simulink model "controlmodel"  (R2016a)
settings: Solver=ode45  StartTime=0.0  StopTime=12.0  RelTol=1e-3
values from neighbouring files (symbols this model uses):
  gainBFL = 1    [LoadModel_dampedTM.m]
  gainBFP = 1    [LoadModel_dampedTM.m]
  gainBFR = 1    [LoadModel_dampedTM.m]
  gainBFT = 1    [LoadModel_dampedTM.m]
  gainBFV = 1    [LoadModel_dampedTM.m]
  gainBFY = 1    [LoadModel_dampedTM.m]
  gainGASBF = 1    [LoadModel_dampedTM.m]
  gainGASF0 = 1    [LoadModel_dampedTM.m]
  gainGASF1 = 1    [LoadModel_dampedTM.m]
  gainGASF2 = 1    [LoadModel_dampedTM.m]
  gainGASF3 = 1    [LoadModel_dampedTM.m]
  gainIML = 1    [LoadModel_dampedTM.m]
  gainIMP = 1    [LoadModel_dampedTM.m]
  gainIMR = 1    [LoadModel_dampedTM.m]
  gainIMT = 1    [LoadModel_dampedTM.m]
  gainIMV = 1    [LoadModel_dampedTM.m]
  gainIMY = 1    [LoadModel_dampedTM.m]
  gainIPL = 1    [LoadModel_dampedTM.m]
  gainIPT = 1    [LoadModel_dampedTM.m]
  gainIPY = 1    [LoadModel_dampedTM.m]
  gainLOCK_IML = 1    [LoadModel_dampedTM.m]
  gainLOCK_IMP = 1    [LoadModel_dampedTM.m]
  gainLOCK_IMY = 1    [LoadModel_dampedTM.m]
  gainMNL = 1    [LoadModel_dampedTM.m]
  gainMNLOCK_L = 1    [LoadModel_dampedTM.m]
  gainMNLOCK_P = 1    [LoadModel_dampedTM.m]
  gainMNLOCK_Y = 1    [LoadModel_dampedTM.m]
  gainMNP = 1    [LoadModel_dampedTM.m]
  gainMNR = 1    [LoadModel_dampedTM.m]
  gainMNT = 1    [LoadModel_dampedTM.m]
  gainMNV = 1    [LoadModel_dampedTM.m]
  gainMNY = 1    [LoadModel_dampedTM.m]
  gainOL_MNP = 1    [LoadModel_dampedTM.m]
  gainOL_MNY = 1    [LoadModel_dampedTM.m]
  gainTML = 1    [LoadModel_dampedTM.m]
  gainTML_LOCK = 0    [LoadModel_dampedTM.m]
  gainTMOL_IML = 1    [LoadModel_dampedTM.m]
  gainTMOL_IMP = 1    [LoadModel_dampedTM.m]
  gainTMOL_IMY = 1    [LoadModel_dampedTM.m]
  gainTMOL_MNL = 1    [LoadModel_dampedTM.m]
  gainTMOL_MNP = 1    [LoadModel_dampedTM.m]
  gainTMOL_MNY = 1    [LoadModel_dampedTM.m]
  gainTMP = 1    [LoadModel_dampedTM.m]
  gainTMY = 1    [LoadModel_dampedTM.m]
  Kopt_angle = 0.1    [LoadModel_dampedTM.m]
  Kopt_len = 0.1    [LoadModel_dampedTM.m]
  optic = 'ETMX'    [LoadModel_dampedTM.m]
undefined symbols (not defined in the file or in its folder): cMat_BF, cMat_IM, cMat_MN, cMat_TM, Filt, gain_actBFGAS, gain_actBFL, gain_actBFP, gain_actBFR, gain_actBFT, gain_actBFV, gain_actBFY, gain_actF0GAS, gain_actF1GAS, gain_actF2GAS, gain_actF3GAS, gain_actIML, gain_actIMP, gain_actIMR, gain_actIMT, gain_actIMV, gain_actIMY, gain_actIPL, gain_actIPT, gain_actIPY, gain_actMNL, gain_actMNP, gain_actMNR, gain_actMNT, gain_actMNV, gain_actMNY, gain_actTML, gain_actTMP, gain_actTMY, SW, sys1
libraries: cstblocks x49, LiveParts x49
(part 1 of 3)
settings Model: Creator=kokioktm  LastModifiedBy=controls
settings DataIOCC: LimitDataPoints=on  SaveFormat=Array
settings DebuggingCC: SolverPrmCheckMsg=warning
settings HardwareCC: ProdBitPerPointer=32  ProdLargestAtomicFloat=None  ProdIntDivRoundTo=Undefined  ProdEndianess=Unspecified  ProdWordSize=32  ProdHWDeviceType=32-bit Generic
settings ModelReferenceCC: PropagateSignalLabelsOutOfModel=off
settings ConfigComp: CovSFcnEnable=off

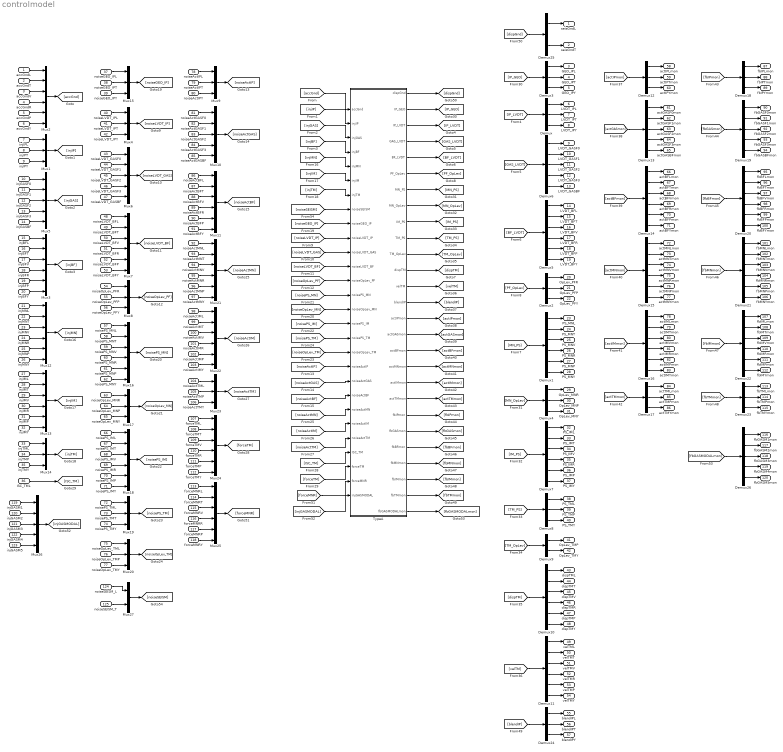
== system controlmodel ==
  accGndL : Inport
  accGndT : Inport  Port=2
  accGndV : Inport  Port=3
  accGndR : Inport  Port=4
  accGndP : Inport  Port=5
  accGndY : Inport  Port=6
  injIPL : Inport  Port=7
  injIPT : Inport  Port=8
  injIPY : Inport  Port=9
  injGASF0 : Inport  Port=10
  injGASF1 : Inport  Port=11
  injGASF2 : Inport  Port=12
  injGASF3 : Inport  Port=13
  injGASBF : Inport  Port=14
  injBFL : Inport  Port=15
  injBFT : Inport  Port=16
  injBFV : Inport  Port=17
  injBFR : Inport  Port=18
  injBFP : Inport  Port=19
  injBFY : Inport  Port=20
  injMNL : Inport  Port=21
  injMNT : Inport  Port=22
  injMNV : Inport  Port=23
  injMNR : Inport  Port=24
  injMNP : Inport  Port=25
  injMNY : Inport  Port=26
  injIML : Inport  Port=27
  injIMT : Inport  Port=28
  injIMV : Inport  Port=29
  injIMR : Inport  Port=30
  injIMP : Inport  Port=31
  injIMY : Inport  Port=32
  injTML : Inport  Port=33
  injTMP : Inport  Port=34
  injTMY : Inport  Port=35
  ISC_TML : Inport  Port=36
  noiseGEO_IPL : Inport  Port=37
  noiseGEO_IPT : Inport  Port=38
  noiseGEO_IPY : Inport  Port=39
  noiseLVDT_IPL : Inport  Port=40
  noiseLVDT_IPT : Inport  Port=41
  noiseLVDT_IPY : Inport  Port=42
  noiseLVDT_GASF0 : Inport  Port=43
  noiseLVDT_GASF1 : Inport  Port=44
  noiseLVDT_GASF2 : Inport  Port=45
  noiseLVDT_GASF3 : Inport  Port=46
  noiseLVDT_GASBF : Inport  Port=47
  noiseLVDT_BFL : Inport  Port=48
  noiseLVDT_BFT : Inport  Port=49
  noiseLVDT_BFV : Inport  Port=50
  noiseLVDT_BFR : Inport  Port=51
  noiseLVDT_BFP : Inport  Port=52
  noiseLVDT_BFY : Inport  Port=53
  noiseOpLev_PFR : Inport  Port=54
  noiseOpLev_PFP : Inport  Port=55
  noiseOpLev_PFY : Inport  Port=56
  noisePS_MNL : Inport  Port=57
  noisePS_MNT : Inport  Port=58
  noisePS_MNV : Inport  Port=59
  noisePS_MNR : Inport  Port=60
  noisePS_MNP : Inport  Port=61
  noisePS_MNY : Inport  Port=62
  noiseOpLev_MNR : Inport  Port=63
  noiseOpLev_MNP : Inport  Port=64
  noiseOpLev_MNY : Inport  Port=65
  noisePS_IML : Inport  Port=66
  noisePS_IMT : Inport  Port=67
  noisePS_IMV : Inport  Port=68
  noisePS_IMR : Inport  Port=69
  noisePS_IMP : Inport  Port=70
  noisePS_IMY : Inport  Port=71
  noisePS_TML : Inport  Port=72
  noisePS_TMT : Inport  Port=73
  noisePS_TMY : Inport  Port=74
  noiseOpLev_TML : Inport  Port=75
  noiseOpLev_TMP : Inport  Port=76
  noiseOpLev_TMY : Inport  Port=77
  noiseActIPL : Inport  Port=78
  noiseActIPT : Inport  Port=79
  noiseActIPY : Inport  Port=80
  noiseActGASF0 : Inport  Port=81
  noiseActGASF1 : Inport  Port=82
  noiseActGASF2 : Inport  Port=83
  noiseActGASF3 : Inport  Port=84
  noiseActGASBF : Inport  Port=85
  noiseActBFL : Inport  Port=86
  noiseActBFT : Inport  Port=87
  noiseActBFV : Inport  Port=88
  noiseActBFR : Inport  Port=89
  noiseActBFP : Inport  Port=90
  noiseActBFY : Inport  Port=91
  noiseActMNL : Inport  Port=92
  noiseActMNT : Inport  Port=93
  noiseActMNV : Inport  Port=94
  noiseActMNR : Inport  Port=95
  noiseActMNP : Inport  Port=96
  noiseActMNY : Inport  Port=97
  noiseActIML : Inport  Port=98
  noiseActIMT : Inport  Port=99
  noiseActIMV : Inport  Port=100
  noiseActIMR : Inport  Port=101
  noiseActIMP : Inport  Port=102
  noiseActIMY : Inport  Port=103
  noiseActTML : Inport  Port=104
  noiseActTMP : Inport  Port=105
  noiseActTMY : Inport  Port=106
  forceTML : Inport  Port=107
  forceTMT : Inport  Port=108
  forceTMV : Inport  Port=109
  forceTMR : Inport  Port=110
  forceTMP : Inport  Port=111
  forceTMY : Inport  Port=112
  forceMNRL : Inport  Port=113
  forceMNRT : Inport  Port=114
  forceMNRV : Inport  Port=115
  forceMNRR : Inport  Port=116
  forceMNRP : Inport  Port=117
  forceMNRY : Inport  Port=118
  injGASM1 : Inport  Port=119
  injGASM2 : Inport  Port=120
  injGASM3 : Inport  Port=121
  injGASM4 : Inport  Port=122
  injGASM5 : Inport  Port=123
  noiseSEISM_L : Inport  Port=124
  noiseSEISM_T : Inport  Port=125
  Demux{,2..4,8,12,17..18,23..24} (10 alike) : Demux  Outputs=3
  Demux{1,5,7,10..11,14..16,20..22} (11 alike) : Demux  Outputs=6
  Demux{6,13,19,26} (4 alike) : Demux  Outputs=5
  Demux25 : Demux  Outputs=2
  Demux9 : Demux  Outputs=2
  Mux{1,4,8..9,14..15,17,19..20,23} (10 alike) : Mux  Inputs=3
  Mux{5..6,10,26} (4 alike) : Mux  Inputs=5
  Mux{2..3,7,11..13,16,18,21..22,24..25} (12 alike) : Mux  Inputs=6
  Mux27 : Mux  Inputs=2
  TypeA : Subsystem
  seisGndL : Outport
  seisGndT : Outport  Port=2
  GEO_IPL : Outport  Port=3
  GEO_IPT : Outport  Port=4
  GEO_IPY : Outport  Port=5
  LVDT_IPL : Outport  Port=6
  LVDT_IPT : Outport  Port=7
  LVDT_IPY : Outport  Port=8
  LVDT_GASF0 : Outport  Port=9
  LVDT_GASF1 : Outport  Port=10
  LVDT_GASF2 : Outport  Port=11
  LVDT_GASF3 : Outport  Port=12
  LVDT_GASBF : Outport  Port=13
  LVDT_BFL : Outport  Port=14
  LVDT_BFT : Outport  Port=15
  LVDT_BFV : Outport  Port=16
  LVDT_BFR : Outport  Port=17
  LVDT_BFP : Outport  Port=18
  LVDT_BFY : Outport  Port=19
  OpLev_PFR : Outport  Port=20
  OpLev_PFP : Outport  Port=21
  OpLev_PFY : Outport  Port=22
  PS_MNL : Outport  Port=23
  PS_MNT : Outport  Port=24
  PS_MNV : Outport  Port=25
  PS_MNR : Outport  Port=26
  PS_MNP : Outport  Port=27
  PS_MNY : Outport  Port=28
  OpLev_MNR : Outport  Port=29
  OpLev_MNP : Outport  Port=30
  OpLev_MNY : Outport  Port=31
  PS_IML : Outport  Port=32
  PS_IMT : Outport  Port=33
  PS_IMV : Outport  Port=34
  PS_IMR : Outport  Port=35
  PS_IMP : Outport  Port=36
  PS_IMY : Outport  Port=37
  PS_TML : Outport  Port=38
  PS_TMP : Outport  Port=39
  PS_TMY : Outport  Port=40
  OpLev_TMP : Outport  Port=41
  OpLev_TMY : Outport  Port=42
  dispTML : Outport  Port=43
  dispTMT : Outport  Port=44
  dispTMV : Outport  Port=45
  dispTMR : Outport  Port=46
  dispTMP : Outport  Port=47
  dispTMY : Outport  Port=48
  velTML : Outport  Port=49
  velTMT : Outport  Port=50
  velTMV : Outport  Port=51
  velTMR : Outport  Port=52
  velTMP : Outport  Port=53
  velTMY : Outport  Port=54
  blendIPL : Outport  Port=55
  blendIPT : Outport  Port=56
  blendIPY : Outport  Port=57
  actIPLmon : Outport  Port=58
  actIPTmon : Outport  Port=59
  actIPYmon : Outport  Port=60
  actGASF0mon : Outport  Port=61
  actGASF1mon : Outport  Port=62
  actGASF2mon : Outport  Port=63
  actGASF3mon : Outport  Port=64
  actGASBFmon : Outport  Port=65
  actBFLmon : Outport  Port=66
  actBFTmon : Outport  Port=67
  actBFVmon : Outport  Port=68
  actBFRmon : Outport  Port=69
  actBFPmon : Outport  Port=70
  actBFYmon : Outport  Port=71
  actMNLmon : Outport  Port=72
  actMNTmon : Outport  Port=73
  actMNVmon : Outport  Port=74
  actMNRmon : Outport  Port=75
  actMNPmon : Outport  Port=76
  actMNYmon : Outport  Port=77
  actIMLmon : Outport  Port=78
  actIMTmon : Outport  Port=79
  actIMVmon : Outport  Port=80
  actIMRmon : Outport  Port=81
  actIMPmon : Outport  Port=82
  actIMYmon : Outport  Port=83
  actTMLmon : Outport  Port=84
  actTMPmon : Outport  Port=85
  actTMYmon : Outport  Port=86
  fbIPLmon : Outport  Port=87
  fbIPTmon : Outport  Port=88
  fbIPYmon : Outport  Port=89
  fbGASF0mon : Outport  Port=90
  fbGASF1mon : Outport  Port=91
  fbGASF2mon : Outport  Port=92
  fbGASF3mon : Outport  Port=93
  fbGASBFmon : Outport  Port=94
  fbBFLmon : Outport  Port=95
  fbBFTmon : Outport  Port=96
  fbBFVmon : Outport  Port=97
  fbBFRmon : Outport  Port=98
  fbBFPmon : Outport  Port=99
  fbBFYmon : Outport  Port=100
  fbMNLmon : Outport  Port=101
  fbMNTmon : Outport  Port=102
  fbMNVmon : Outport  Port=103
  fbMNRmon : Outport  Port=104
  fbMNPmon : Outport  Port=105
  fbMNYmon : Outport  Port=106
  fbIMLmon : Outport  Port=107
  fbIMTmon : Outport  Port=108
  fbIMVmon : Outport  Port=109
  fbIMRmon : Outport  Port=110
  fbIMPmon : Outport  Port=111
  fbIMYmon : Outport  Port=112
  fbTMLmon : Outport  Port=113
  fbTMPmon : Outport  Port=114
  fbTMYmon : Outport  Port=115
  fbGASM1mon : Outport  Port=116
  fbGASM2mon : Outport  Port=117
  fbGASM3mon : Outport  Port=118
  fbGASM4mon : Outport  Port=119
  fbGASM5mon : Outport  Port=120
  wires:
  [accGnd] -> TypeA/1(accGnd)
  accGndT/1 -> Mux2/2
  accGndL/1 -> Mux2/1
  accGndV/1 -> Mux2/3
  accGndR/1 -> Mux2/4
  accGndP/1 -> Mux2/5
  accGndY/1 -> Mux2/6
  Mux2/1 -> [accGnd]
  injIPL/1 -> Mux1/1
  injIPT/1 -> Mux1/2
  injIPY/1 -> Mux1/3
  Mux1/1 -> [injIP]
  [injIP] -> TypeA/2(injIP)
  injGASF0/1 -> Mux5/1
  injGASF1/1 -> Mux5/2
  injGASF2/1 -> Mux5/3
  injGASF3/1 -> Mux5/4
  injGASBF/1 -> Mux5/5
  Mux5/1 -> [injGAS]
  [injGAS] -> TypeA/3(injGAS)
  injBFT/1 -> Mux3/2
  injBFL/1 -> Mux3/1
  injBFV/1 -> Mux3/3
  injBFR/1 -> Mux3/4
  injBFP/1 -> Mux3/5
  injBFY/1 -> Mux3/6
  Mux3/1 -> [injBF]
  [injBF] -> TypeA/4(injBF)
  TypeA/3(IP_LVDT) -> [IP_LVDT]
  TypeA/4(GAS_LVDT) -> [GAS_LVDT]
  TypeA/5(BF_LVDT) -> [BF_LVDT]
  TypeA/12(dispTM) -> [dispTM]
  TypeA/6(PF_OpLev) -> [PF_OpLev]
  [IP_LVDT] -> Demux/1
  Demux/1 -> LVDT_IPL/1
  Demux/2 -> LVDT_IPT/1
  Demux/3 -> LVDT_IPY/1
  [GAS_LVDT] -> Demux6/1
  Demux6/1 -> LVDT_GASF0/1
  Demux6/2 -> LVDT_GASF1/1
  Demux6/3 -> LVDT_GASF2/1
  Demux6/4 -> LVDT_GASF3/1
  Demux6/5 -> LVDT_GASBF/1
  [BF_LVDT] -> Demux5/1
  Demux5/1 -> LVDT_BFL/1
  Demux5/2 -> LVDT_BFT/1
  Demux5/3 -> LVDT_BFV/1
  Demux5/4 -> LVDT_BFR/1
  Demux5/5 -> LVDT_BFP/1
  Demux5/6 -> LVDT_BFY/1
  Demux1/1 -> PS_MNL/1
  Demux1/2 -> PS_MNT/1
  Demux1/3 -> PS_MNV/1
  Demux1/4 -> PS_MNR/1
  Demux1/5 -> PS_MNP/1
  Demux1/6 -> PS_MNY/1
  [MN_PS] -> Demux1/1
  [PF_OpLev] -> Demux2/1
  Demux2/2 -> OpLev_PFP/1
  Demux2/3 -> OpLev_PFY/1
  noiseLVDT_IPL/1 -> Mux4/1
  noiseLVDT_IPT/1 -> Mux4/2
  noiseLVDT_IPY/1 -> Mux4/3
  Mux4/1 -> [noiseLVDT_IP]
  noiseLVDT_GASF0/1 -> Mux6/1
  noiseLVDT_GASF1/1 -> Mux6/2
  noiseLVDT_GASF2/1 -> Mux6/3
  noiseLVDT_GASF3/1 -> Mux6/4
  noiseLVDT_GASBF/1 -> Mux6/5
  Mux6/1 -> [noiseLVDT_GAS]
  noiseLVDT_BFT/1 -> Mux7/2
  noiseLVDT_BFL/1 -> Mux7/1
  noiseLVDT_BFV/1 -> Mux7/3
  noiseLVDT_BFR/1 -> Mux7/4
  noiseLVDT_BFP/1 -> Mux7/5
  noiseLVDT_BFY/1 -> Mux7/6
  Mux7/1 -> [noiseLVDT_BF]
  noiseOpLev_PFR/1 -> Mux8/1
  noiseOpLev_PFP/1 -> Mux8/2
  Mux8/1 -> [noiseOpLev_PF]
  [noiseLVDT_IP] -> TypeA/10(noiseLVDT_IP)
  [noiseLVDT_GAS] -> TypeA/11(noiseLVDT_GAS)
  [noiseOpLev_PF] -> TypeA/13(noiseOpLev_PF)
  [noiseLVDT_BF] -> TypeA/12(noiseLVDT_BF)
  noiseActIPL/1 -> Mux9/1
  noiseActIPT/1 -> Mux9/2
  noiseActIPY/1 -> Mux9/3
  Mux9/1 -> [noiseActIP]
  noiseActGASF0/1 -> Mux10/1
  noiseActGASF1/1 -> Mux10/2
  noiseActGASF2/1 -> Mux10/3
  noiseActGASF3/1 -> Mux10/4
  noiseActGASBF/1 -> Mux10/5
  Mux10/1 -> [noiseActGAS]
  noiseActBFT/1 -> Mux11/2
  noiseActBFL/1 -> Mux11/1
  noiseActBFV/1 -> Mux11/3
  noiseActBFR/1 -> Mux11/4
  noiseActBFP/1 -> Mux11/5
  noiseActBFY/1 -> Mux11/6
  Mux11/1 -> [noiseActBF]
  [noiseActGAS] -> TypeA/20(noiseActGAS)
  [noiseActBF] -> TypeA/21(noiseActBF)
  [noiseActIP] -> TypeA/19(noiseActIP)
  [injMN] -> TypeA/5(injMN)
  [injTM] -> TypeA/7(injTM)
  [injIM] -> TypeA/6(injIM)
  injMNT/1 -> Mux12/2
  injMNL/1 -> Mux12/1
  injMNV/1 -> Mux12/3
  injMNR/1 -> Mux12/4
  injMNP/1 -> Mux12/5
  injMNY/1 -> Mux12/6
  Mux12/1 -> [injMN]
  injIMT/1 -> Mux13/2
  injIML/1 -> Mux13/1
  injIMV/1 -> Mux13/3
  injIMR/1 -> Mux13/4
  injIMP/1 -> Mux13/5
  injIMY/1 -> Mux13/6
  Mux13/1 -> [injIM]
  injTML/1 -> Mux14/1
  injTMP/1 -> Mux14/2
  injTMY/1 -> Mux14/3
  Mux14/1 -> [injTM]
  noiseGEO_IPL/1 -> Mux15/1
  noiseGEO_IPT/1 -> Mux15/2
  noiseGEO_IPY/1 -> Mux15/3
  Mux15/1 -> [noiseGEO_IP]
  [noiseGEO_IP] -> TypeA/9(noiseGEO_IP)
  noiseOpLev_PFY/1 -> Mux8/3
  noisePS_MNT/1 -> Mux16/2
  noisePS_MNL/1 -> Mux16/1
  noisePS_MNV/1 -> Mux16/3
  noisePS_MNR/1 -> Mux16/4
  noisePS_MNP/1 -> Mux16/5
  noisePS_MNY/1 -> Mux16/6
  Mux16/1 -> [noisePS_MN]
  noiseOpLev_MNR/1 -> Mux17/1
  noiseOpLev_MNP/1 -> Mux17/2
  Mux17/1 -> [noiseOpLev_MN]
  noiseOpLev_MNY/1 -> Mux17/3
  noisePS_IMT/1 -> Mux18/2
  noisePS_IML/1 -> Mux18/1
  noisePS_IMV/1 -> Mux18/3
  noisePS_IMR/1 -> Mux18/4
  noisePS_IMP/1 -> Mux18/5
  noisePS_IMY/1 -> Mux18/6
  Mux18/1 -> [noisePS_IM]
  noisePS_TML/1 -> Mux19/1
  noisePS_TMT/1 -> Mux19/2
  Mux19/1 -> [noisePS_TM]
  noisePS_TMY/1 -> Mux19/3
  noiseOpLev_TMP/1 -> Mux20/2
  noiseOpLev_TMY/1 -> Mux20/3
  Mux20/1 -> [noiseOpLev_TM]
  [noisePS_MN] -> TypeA/14(noisePS_MN)
  [noisePS_IM] -> TypeA/16(noisePS_IM)
  [noiseOpLev_MN] -> TypeA/15(noiseOpLev_MN)
  [noisePS_TM] -> TypeA/17(noisePS_TM)
  [noiseOpLev_TM] -> TypeA/18(noiseOpLev_TM)
  noiseActMNT/1 -> Mux21/2
  noiseActMNL/1 -> Mux21/1
  noiseActMNV/1 -> Mux21/3
  noiseActMNR/1 -> Mux21/4
  noiseActMNP/1 -> Mux21/5
  noiseActMNY/1 -> Mux21/6
  Mux21/1 -> [noiseActMN]
  noiseActIMT/1 -> Mux22/2
  noiseActIML/1 -> Mux22/1
  noiseActIMV/1 -> Mux22/3
  noiseActIMR/1 -> Mux22/4
  noiseActIMP/1 -> Mux22/5
  noiseActIMY/1 -> Mux22/6
  Mux22/1 -> [noiseActIM]
  noiseActTML/1 -> Mux23/1
  noiseActTMP/1 -> Mux23/2
  noiseActTMY/1 -> Mux23/3
  Mux23/1 -> [noiseActTM]
  forceTMT/1 -> Mux24/2
  forceTML/1 -> Mux24/1
  forceTMV/1 -> Mux24/3
  forceTMR/1 -> Mux24/4
  forceTMP/1 -> Mux24/5
  forceTMY/1 -> Mux24/6
  Mux24/1 -> [forceTM]
  ISC_TML/1 -> [ISC_TM]
  [noiseActMN] -> TypeA/22(noiseActMN)
  [noiseActTM] -> TypeA/24(noiseActTM)
  [noiseActIM] -> TypeA/23(noiseActIM)
  [forceTM] -> TypeA/26(forceTM)
  [ISC_TM] -> TypeA/25(ISC_TM)
  [IP_GEO] -> Demux3/1
  Demux3/1 -> GEO_IPL/1
  Demux3/2 -> GEO_IPT/1
  Demux3/3 -> GEO_IPY/1
  TypeA/2(IP_GEO) -> [IP_GEO]
  Demux2/1 -> OpLev_PFR/1
  TypeA/9(IM_PS) -> [IM_PS]
  TypeA/10(TM_PS) -> [TM_PS]
  TypeA/8(MN_OpLev) -> [MN_OpLev]
  TypeA/7(MN_PS) -> [MN_PS]
  TypeA/11(TM_OpLev) -> [TM_OpLev]
  TypeA/22(fbGASmon) -> [fbGASmon]
  TypeA/16(actGASmon) -> [actGASmon]
  TypeA/21(fbIPmon) -> [fbIPmon]
  TypeA/26(fbTMmon) -> [fbTMmon]
  TypeA/24(fbMNmon) -> [fbMNmon]
  TypeA/15(actIPmon) -> [actIPmon]
  TypeA/19(actIMmon) -> [actIMmon]
  TypeA/14(blendIP) -> [blendIP]
  TypeA/13(velTM) -> [velTM]
  TypeA/25(fbIMmon) -> [fbIMmon]
  TypeA/18(actMNmon) -> [actMNmon]
  TypeA/20(actTMmon) -> [actTMmon]
  TypeA/17(actBFmon) -> [actBFmon]
  TypeA/23(fbBFmon) -> [fbBFmon]
  [MN_OpLev] -> Demux4/1
  Demux4/2 -> OpLev_MNP/1
  Demux4/3 -> OpLev_MNY/1
  Demux4/1 -> OpLev_MNR/1
  Demux7/1 -> PS_IML/1
  Demux7/2 -> PS_IMT/1
  Demux7/3 -> PS_IMV/1
  Demux7/4 -> PS_IMR/1
  Demux7/5 -> PS_IMP/1
  Demux7/6 -> PS_IMY/1
  [IM_PS] -> Demux7/1
  Demux8/1 -> PS_TML/1
  [TM_PS] -> Demux8/1
  Demux8/2 -> PS_TMP/1
  Demux8/3 -> PS_TMY/1
  [TM_OpLev] -> Demux9/1
  Demux9/1 -> OpLev_TMP/1
  Demux9/2 -> OpLev_TMY/1
  Demux10/1 -> dispTML/1
  Demux10/2 -> dispTMT/1
  Demux10/3 -> dispTMV/1
  Demux10/4 -> dispTMR/1
  Demux10/5 -> dispTMP/1
  Demux10/6 -> dispTMY/1
  [dispTM] -> Demux10/1
  Demux11/1 -> velTML/1
  Demux11/2 -> velTMT/1
  Demux11/3 -> velTMV/1
  Demux11/4 -> velTMR/1
  Demux11/5 -> velTMP/1
  Demux11/6 -> velTMY/1
  [velTM] -> Demux11/1
  [actIPmon] -> Demux12/1
  Demux12/1 -> actIPLmon/1
  Demux12/2 -> actIPTmon/1
  Demux12/3 -> actIPYmon/1
  [actGASmon] -> Demux13/1
  Demux13/1 -> actGASF0mon/1
  Demux13/2 -> actGASF1mon/1
  Demux13/3 -> actGASF2mon/1
  Demux13/4 -> actGASF3mon/1
  Demux13/5 -> actGASBFmon/1
  [actBFmon] -> Demux14/1
  Demux14/1 -> actBFLmon/1
  Demux14/2 -> actBFTmon/1
  Demux14/3 -> actBFVmon/1
  Demux14/4 -> actBFRmon/1
  Demux14/5 -> actBFPmon/1
  Demux14/6 -> actBFYmon/1
  [actMNmon] -> Demux15/1
  Demux15/1 -> actMNLmon/1
  Demux15/2 -> actMNTmon/1
  Demux15/3 -> actMNVmon/1
  Demux15/4 -> actMNRmon/1
  Demux15/5 -> actMNPmon/1
  Demux15/6 -> actMNYmon/1
  [actIMmon] -> Demux16/1
  Demux16/1 -> actIMLmon/1
  Demux16/2 -> actIMTmon/1
  Demux16/3 -> actIMVmon/1
  Demux16/4 -> actIMRmon/1
  Demux16/5 -> actIMPmon/1
  Demux16/6 -> actIMYmon/1
  [actTMmon] -> Demux17/1
  Demux17/2 -> actTMPmon/1
  Demux17/3 -> actTMYmon/1
  Demux17/1 -> actTMLmon/1
  [fbIPmon] -> Demux18/1
  Demux18/1 -> fbIPLmon/1
  Demux18/2 -> fbIPTmon/1
  Demux18/3 -> fbIPYmon/1
  [fbGASmon] -> Demux19/1
  Demux19/1 -> fbGASF0mon/1
  Demux19/2 -> fbGASF1mon/1
  Demux19/3 -> fbGASF2mon/1
  Demux19/4 -> fbGASF3mon/1
  Demux19/5 -> fbGASBFmon/1
  [fbBFmon] -> Demux20/1
  Demux20/1 -> fbBFLmon/1
  Demux20/2 -> fbBFTmon/1
  Demux20/3 -> fbBFVmon/1
  Demux20/4 -> fbBFRmon/1
  Demux20/5 -> fbBFPmon/1
  Demux20/6 -> fbBFYmon/1
  [fbMNmon] -> Demux21/1
  Demux21/1 -> fbMNLmon/1
  Demux21/2 -> fbMNTmon/1
  Demux21/3 -> fbMNVmon/1
  Demux21/4 -> fbMNRmon/1
  Demux21/5 -> fbMNPmon/1
  Demux21/6 -> fbMNYmon/1
  [fbIMmon] -> Demux22/1
  Demux22/1 -> fbIMLmon/1
  Demux22/2 -> fbIMTmon/1
  Demux22/3 -> fbIMVmon/1
  Demux22/4 -> fbIMRmon/1
  Demux22/5 -> fbIMPmon/1
  Demux22/6 -> fbIMYmon/1
  [fbTMmon] -> Demux23/1
  Demux23/2 -> fbTMPmon/1
  Demux23/3 -> fbTMYmon/1
  Demux23/1 -> fbTMLmon/1
  Demux24/1 -> blendIPL/1
  [blendIP] -> Demux24/1
  Demux24/2 -> blendIPT/1
  Demux24/3 -> blendIPY/1
  [dispGnd] -> Demux25/1
  Demux25/1 -> seisGndL/1
  Demux25/2 -> seisGndT/1
  TypeA/1(dispGnd) -> [dispGnd]
  forceMNRR/1 -> Mux25/4
  forceMNRP/1 -> Mux25/5
  forceMNRL/1 -> Mux25/1
  forceMNRT/1 -> Mux25/2
  Mux25/1 -> [forceMNR]
  forceMNRV/1 -> Mux25/3
  forceMNRY/1 -> Mux25/6
  [forceMNR] -> TypeA/27(forceMNR)
  noiseOpLev_TML/1 -> Mux20/1
  [injGASMODAL] -> TypeA/28(injGASMODAL)
  injGASM1/1 -> Mux26/1
  injGASM2/1 -> Mux26/2
  injGASM3/1 -> Mux26/3
  injGASM4/1 -> Mux26/4
  injGASM5/1 -> Mux26/5
  Mux26/1 -> [injGASMODAL]
  TypeA/27(fbGASMODALmon) -> [fbGASMODALmon]
  [fbGASMODALmon] -> Demux26/1
  Demux26/1 -> fbGASM1mon/1
  Demux26/2 -> fbGASM2mon/1
  Demux26/3 -> fbGASM3mon/1
  Demux26/4 -> fbGASM4mon/1
  Demux26/5 -> fbGASM5mon/1
  [noiseSEISM] -> TypeA/8(noiseSEISM)
  noiseSEISM_T/1 -> Mux27/2
  Mux27/1 -> [noiseSEISM]
  noiseSEISM_L/1 -> Mux27/1

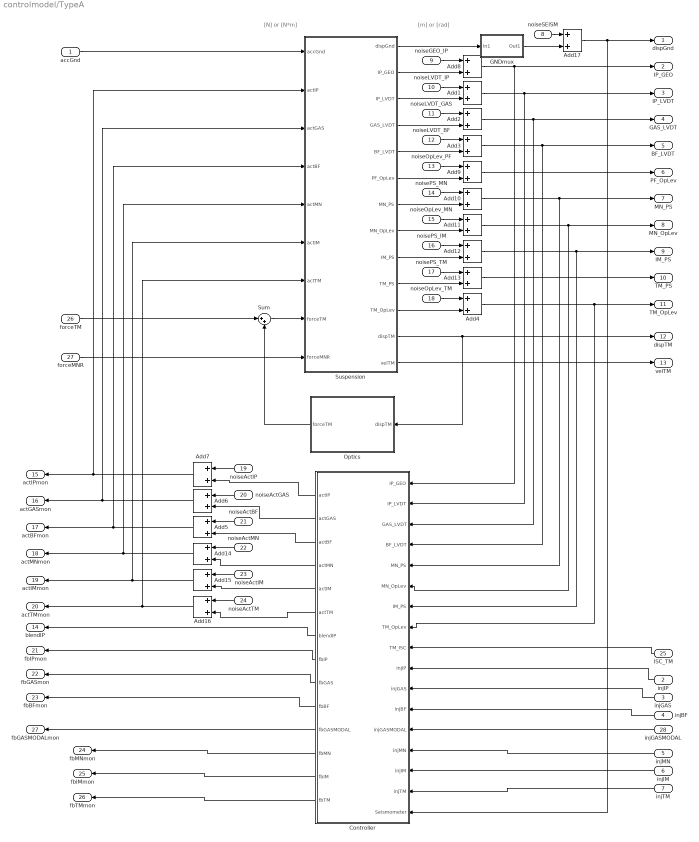
== system controlmodel/TypeA ==
  note: [N] or [N*m]
  note: [m] or [rad]
  accGnd : Inport
  injIP : Inport  Port=2
  injGAS : Inport  Port=3
  injBF : Inport  Port=4
  injMN : Inport  Port=5
  injIM : Inport  Port=6
  injTM : Inport  Port=7
  noiseSEISM : Inport  Port=8
  noiseGEO_IP : Inport  Port=9
  noiseLVDT_IP : Inport  Port=10
  noiseLVDT_GAS : Inport  Port=11
  noiseLVDT_BF : Inport  Port=12
  noiseOpLev_PF : Inport  Port=13
  noisePS_MN : Inport  Port=14
  noiseOpLev_MN : Inport  Port=15
  noisePS_IM : Inport  Port=16
  noisePS_TM : Inport  Port=17
  noiseOpLev_TM : Inport  Port=18
  noiseActIP : Inport  Port=19
  noiseActGAS : Inport  Port=20
  noiseActBF : Inport  Port=21
  noiseActMN : Inport  Port=22
  noiseActIM : Inport  Port=23
  noiseActTM : Inport  Port=24
  ISC_TM : Inport  Port=25
  forceTM : Inport  Port=26
  forceMNR : Inport  Port=27
  injGASMODAL : Inport  Port=28
  Add{1..17} (17 alike) : Sum
  Controller : Subsystem
  GNDmux : Subsystem
  Optics : Subsystem
  Sum : Sum  Inputs=|++
  Suspension : Subsystem
  dispGnd : Outport
  IP_GEO : Outport  Port=2
  IP_LVDT : Outport  Port=3
  GAS_LVDT : Outport  Port=4
  BF_LVDT : Outport  Port=5
  PF_OpLev : Outport  Port=6
  MN_PS : Outport  Port=7
  MN_OpLev : Outport  Port=8
  IM_PS : Outport  Port=9
  TM_PS : Outport  Port=10
  TM_OpLev : Outport  Port=11
  dispTM : Outport  Port=12
  velTM : Outport  Port=13
  blendIP : Outport  Port=14
  actIPmon : Outport  Port=15
  actGASmon : Outport  Port=16
  actBFmon : Outport  Port=17
  actMNmon : Outport  Port=18
  actIMmon : Outport  Port=19
  actTMmon : Outport  Port=20
  fbIPmon : Outport  Port=21
  fbGASmon : Outport  Port=22
  fbBFmon : Outport  Port=23
  fbMNmon : Outport  Port=24
  fbIMmon : Outport  Port=25
  fbTMmon : Outport  Port=26
  fbGASMODALmon : Outport  Port=27
  wires:
  Add1/1 -> IP_LVDT/1, Controller/2(IP_LVDT)
  Add3/1 -> Controller/4(BF_LVDT), BF_LVDT/1
  Add2/1 -> GAS_LVDT/1, Controller/3(GAS_LVDT)
  Add7/1 -> actIPmon/1, Suspension/2(actIP)
  Add5/1 -> actBFmon/1, Suspension/4(actBF)
  Add4/1 -> Controller/8(TM_OpLev), TM_OpLev/1
  accGnd/1 -> Suspension/1(accGnd)
  Add6/1 -> actGASmon/1, Suspension/3(actGAS)
  injGAS/1 -> Controller/11(injGAS)
  injIP/1 -> Controller/10(injIP)
  injBF/1 -> Controller/12(injBF)
  Controller/10(fbBF) -> fbBFmon/1
  Controller/8(fbIP) -> fbIPmon/1
  Controller/9(fbGAS) -> fbGASmon/1
  Suspension/3(IP_LVDT) -> Add1/2
  Suspension/4(GAS_LVDT) -> Add2/2
  Suspension/5(BF_LVDT) -> Add3/2
  Suspension/11(TM_OpLev) -> Add4/2
  noiseLVDT_IP/1 -> Add1/1
  noiseLVDT_GAS/1 -> Add2/1
  noiseLVDT_BF/1 -> Add3/1
  noiseOpLev_TM/1 -> Add4/1
  Controller/3(actBF) -> Add5/2
  Controller/1(actIP) -> Add7/2
  Controller/2(actGAS) -> Add6/2
  noiseActIP/1 -> Add7/1
  noiseActGAS/1 -> Add6/1
  noiseActBF/1 -> Add5/1
  Add8/1 -> Controller/1(IP_GEO), IP_GEO/1
  noiseGEO_IP/1 -> Add8/1
  Suspension/2(IP_GEO) -> Add8/2
  noiseOpLev_PF/1 -> Add9/1
  Suspension/6(PF_OpLev) -> Add9/2
  Add9/1 -> PF_OpLev/1
  noisePS_MN/1 -> Add10/1
  Add10/1 -> Controller/5(MN_PS), MN_PS/1
  noiseOpLev_MN/1 -> Add11/1
  Add11/1 -> Controller/6(MN_OpLev), MN_OpLev/1
  noisePS_IM/1 -> Add12/1
  Add12/1 -> Controller/7(IM_PS), IM_PS/1
  Suspension/8(MN_OpLev) -> Add11/2
  Suspension/7(MN_PS) -> Add10/2
  Suspension/9(IM_PS) -> Add12/2
  noisePS_TM/1 -> Add13/1
  Add13/1 -> TM_PS/1
  Suspension/10(TM_PS) -> Add13/2
  Suspension/13(velTM) -> velTM/1
  injMN/1 -> Controller/14(injMN)
  injTM/1 -> Controller/16(injTM)
  injIM/1 -> Controller/15(injIM)
  ISC_TM/1 -> Controller/9(TM_ISC)
  noiseActMN/1 -> Add14/1
  Add14/1 -> Suspension/5(actMN), actMNmon/1
  Controller/4(actMN) -> Add14/2
  noiseActIM/1 -> Add15/1
  Add15/1 -> Suspension/6(actIM), actIMmon/1
  Controller/5(actIM) -> Add15/2
  noiseActTM/1 -> Add16/1
  Add16/1 -> Suspension/7(actTM), actTMmon/1
  Controller/6(actTM) -> Add16/2
  Controller/7(blendIP) -> blendIP/1
  Controller/14(fbTM) -> fbTMmon/1
  Controller/12(fbMN) -> fbMNmon/1
  Controller/13(fbIM) -> fbIMmon/1
  forceMNR/1 -> Suspension/9(forceMNR)
  injGASMODAL/1 -> Controller/13(injGASMODAL)
  Controller/11(fbGASMODAL) -> fbGASMODALmon/1
  noiseSEISM/1 -> Add17/1
  Add17/1 -> Controller/17(Seismometer), dispGnd/1
  Suspension/12(dispTM) -> Optics/1(dispTM), dispTM/1
  Optics/1(forceTM) -> Sum/2
  forceTM/1 -> Sum/1
  Sum/1 -> Suspension/8(forceTM)
  Suspension/1(dispGnd) -> GNDmux/1(In1)
  GNDmux/1(Out1) -> Add17/2

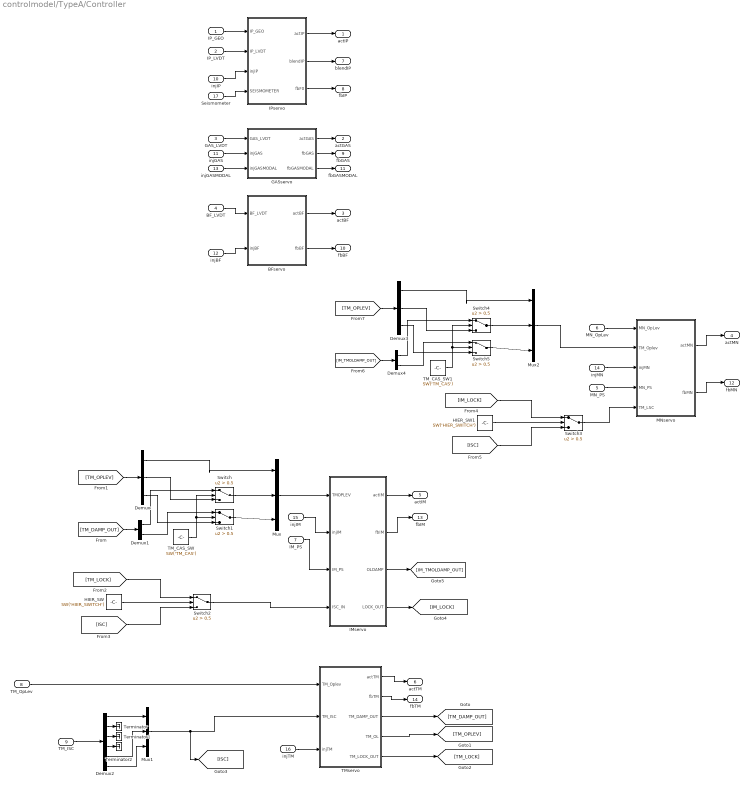
== system controlmodel/TypeA/Controller ==
  IP_GEO : Inport
  IP_LVDT : Inport  Port=2
  GAS_LVDT : Inport  Port=3
  BF_LVDT : Inport  Port=4
  MN_PS : Inport  Port=5
  MN_OpLev : Inport  Port=6
  IM_PS : Inport  Port=7
  TM_OpLev : Inport  Port=8
  TM_ISC : Inport  Port=9
  injIP : Inport  Port=10
  injGAS : Inport  Port=11
  injBF : Inport  Port=12
  injGASMODAL : Inport  Port=13
  injMN : Inport  Port=14
  injIM : Inport  Port=15
  injTM : Inport  Port=16
  Seismometer : Inport  Port=17
  BFservo : Subsystem
  Demux : Demux  Outputs=3
  Demux1 : Demux  Outputs=2
  Demux2 : Demux  Outputs=6
  Demux3 : Demux  Outputs=3
  Demux4 : Demux  Outputs=2
  GASservo : Subsystem
  HIER_SW : Constant  Value=SW('HIER_SWITCH')
  HIER_SW1 : Constant  Value=SW('HIER_SWITCH')
  IMservo : Subsystem
  IPservo : Subsystem
  MNservo : Subsystem
  Mux : Mux  Inputs=3
  Mux1 : Mux  Inputs=3
  Mux2 : Mux  Inputs=3
  Switch{,1..5} (6 alike) : Switch  Criteria=u2 > Threshold  Threshold=0.5
  TM_CAS_SW : Constant  Value=SW('TM_CAS')
  TM_CAS_SW1 : Constant  Value=SW('TM_CAS')
  TMservo : Subsystem
  Terminator : Terminator
  Terminator1 : Terminator
  Terminator2 : Terminator
  actIP : Outport
  actGAS : Outport  Port=2
  actBF : Outport  Port=3
  actMN : Outport  Port=4
  actIM : Outport  Port=5
  actTM : Outport  Port=6
  blendIP : Outport  Port=7
  fbIP : Outport  Port=8
  fbGAS : Outport  Port=9
  fbBF : Outport  Port=10
  fbGASMODAL : Outport  Port=11
  fbMN : Outport  Port=12
  fbIM : Outport  Port=13
  fbTM : Outport  Port=14
  wires:
  IP_LVDT/1 -> IPservo/2(IP_LVDT)
  injIP/1 -> IPservo/3(injIP)
  IPservo/3(fbF0) -> fbIP/1
  IPservo/1(actIP) -> actIP/1
  GASservo/1(actGAS) -> actGAS/1
  GASservo/2(fbGAS) -> fbGAS/1
  GAS_LVDT/1 -> GASservo/1(GAS_LVDT)
  injGAS/1 -> GASservo/2(injGAS)
  BF_LVDT/1 -> BFservo/1(BF_LVDT)
  injBF/1 -> BFservo/2(injBF)
  BFservo/1(actBF) -> actBF/1
  BFservo/2(fbBF) -> fbBF/1
  IP_GEO/1 -> IPservo/1(IP_GEO)
  IPservo/2(blendIP) -> blendIP/1
  TM_OpLev/1 -> TMservo/1(TM_Oplev)
  injGASMODAL/1 -> GASservo/3(injGASMODAL)
  GASservo/3(fbGASMODAL) -> fbGASMODAL/1
  injTM/1 -> TMservo/3(injTM)
  MN_OpLev/1 -> MNservo/1(MN_OpLev)
  injMN/1 -> MNservo/3(injMN)
  injIM/1 -> IMservo/2(injIM)
  TMservo/1(actTM) -> actTM/1
  TMservo/2(fbTM) -> fbTM/1
  IMservo/2(fbIM) -> fbIM/1
  IMservo/1(actIM) -> actIM/1
  MNservo/2(fbMN) -> fbMN/1
  MNservo/1(actMN) -> actMN/1
  MN_PS/1 -> MNservo/4(MN_PS)
  IM_PS/1 -> IMservo/3(IM_PS)
  TMservo/3(TM_DAMP_OUT) -> [TM_DAMP_OUT]
  TM_CAS_SW/1 -> Switch1/2, Switch/2
  [TM_OPLEV] -> Demux/1
  Demux/1 -> Mux/1
  Mux/1 -> IMservo/1(TMOPLEV)
  Switch/1 -> Mux/2
  Switch1/1 -> Mux/3
  Demux/2 -> Switch/3
  Demux/3 -> Switch1/3
  Demux1/1 -> Switch/1
  Demux1/2 -> Switch1/1
  [TM_DAMP_OUT] -> Demux1/1
  TMservo/4(TM_OL) -> [TM_OPLEV]
  Mux1/1 -> [ISC], TMservo/2(TM_ISC)
  TM_ISC/1 -> Demux2/1
  Demux2/1 -> Mux1/1
  Demux2/5 -> Mux1/2
  Demux2/6 -> Mux1/3
  Demux2/2 -> Terminator/1
  Demux2/3 -> Terminator1/1
  Demux2/4 -> Terminator2/1
  TMservo/5(TM_LOCK_OUT) -> [TM_LOCK]
  HIER_SW/1 -> Switch2/2
  [ISC] -> Switch2/3
  [TM_LOCK] -> Switch2/1
  Switch2/1 -> IMservo/4(ISC_IN)
  IMservo/4(LOCK_OUT) -> [IM_LOCK]
  HIER_SW1/1 -> Switch3/2
  [ISC] -> Switch3/3
  [IM_LOCK] -> Switch3/1
  Switch3/1 -> MNservo/5(TM_LSC)
  TM_CAS_SW1/1 -> Switch5/2, Switch4/2
  [TM_OPLEV] -> Demux3/1
  Demux3/1 -> Mux2/1
  Switch4/1 -> Mux2/2
  Switch5/1 -> Mux2/3
  Demux3/2 -> Switch4/3
  Demux3/3 -> Switch5/3
  Demux4/1 -> Switch4/1
  Demux4/2 -> Switch5/1
  [IM_TMOLDAMP_OUT] -> Demux4/1
  IMservo/3(OLDAMP) -> [IM_TMOLDAMP_OUT]
  Mux2/1 -> MNservo/2(TM_Oplev)
  Seismometer/1 -> IPservo/4(SEISMOMETER)

== system controlmodel/TypeA/GNDmux ==
  In1 : Inport
  Demux : Demux
  Mux : Mux  Inputs=2
  Terminator : Terminator
  Terminator1 : Terminator
  Out1 : Outport
  wires:
  Mux/1 -> Out1/1
  Demux/4 -> Terminator/1  "Y"
  Demux/1 -> Mux/1  "L"
  Demux/3 -> Terminator1/1  "V"
  In1/1 -> Demux/1
  Demux/2 -> Mux/2  "T"

== system controlmodel/TypeA/Optics ==
  dispTM : Inport
  Demux : Demux  Outputs=6
  Ground : Ground
  Kopt_angle : Gain  Gain=Kopt_angle
  Kopt_angle1 : Gain  Gain=Kopt_angle
  Kopt_len : Gain  Gain=Kopt_len
  Mux : Mux  Inputs=6
  Terminator1 : Terminator
  Terminator2 : Terminator
  Terminator3 : Terminator
  forceTM : Outport
  wires:
  dispTM/1 -> Demux/1
  Demux/6 -> Kopt_angle1/1
  Kopt_angle1/1 -> Mux/6
  Demux/5 -> Kopt_angle/1
  Kopt_angle/1 -> Mux/5
  Demux/2 -> Terminator1/1
  Demux/3 -> Terminator2/1
  Demux/4 -> Terminator3/1
  Mux/1 -> forceTM/1
  Demux/1 -> Kopt_len/1
  Kopt_len/1 -> Mux/1
  Ground/1 -> Mux/4, Mux/3, Mux/2

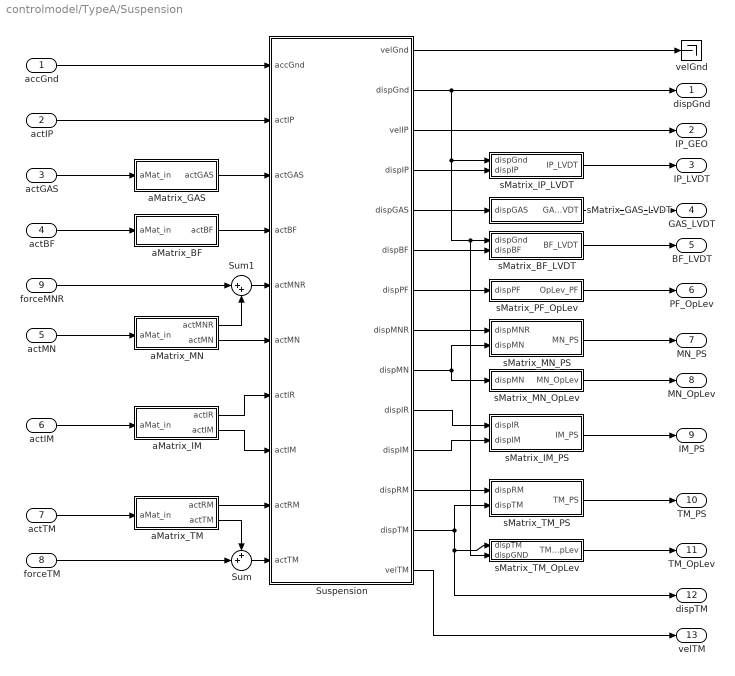
== system controlmodel/TypeA/Suspension ==
  accGnd : Inport
  actIP : Inport  Port=2
  actGAS : Inport  Port=3
  actBF : Inport  Port=4
  actMN : Inport  Port=5
  actIM : Inport  Port=6
  actTM : Inport  Port=7
  forceTM : Inport  Port=8
  forceMNR : Inport  Port=9
  Sum : Sum  Inputs=++|
  Sum1 : Sum  Inputs=|++
  Suspension : Subsystem
  aMatrix_BF : Subsystem
  aMatrix_GAS : Subsystem
  aMatrix_IM : Subsystem
  aMatrix_MN : Subsystem
  aMatrix_TM : Subsystem
  sMatrix_BF_LVDT : Subsystem
  sMatrix_GAS_LVDT : Subsystem
  sMatrix_IM_PS : Subsystem
  sMatrix_IP_LVDT : Subsystem
  sMatrix_MN_OpLev : Subsystem
  sMatrix_MN_PS : Subsystem
  sMatrix_PF_OpLev : Subsystem
  sMatrix_TM_OpLev : Subsystem
  sMatrix_TM_PS : Subsystem
  velGnd : Terminator
  dispGnd : Outport
  IP_GEO : Outport  Port=2
  IP_LVDT : Outport  Port=3
  GAS_LVDT : Outport  Port=4
  BF_LVDT : Outport  Port=5
  PF_OpLev : Outport  Port=6
  MN_PS : Outport  Port=7
  MN_OpLev : Outport  Port=8
  IM_PS : Outport  Port=9
  TM_PS : Outport  Port=10
  TM_OpLev : Outport  Port=11
  dispTM : Outport  Port=12
  velTM : Outport  Port=13
  wires:
  Suspension/2(dispGnd) -> dispGnd/1, sMatrix_TM_OpLev/2(dispGND), sMatrix_BF_LVDT/1(dispGnd), sMatrix_IP_LVDT/1(dispGnd)
  Suspension/4(dispIP) -> sMatrix_IP_LVDT/2(dispIP)
  Suspension/5(dispGAS) -> sMatrix_GAS_LVDT/1(dispGAS)
  Suspension/6(dispBF) -> sMatrix_BF_LVDT/2(dispBF)
  Suspension/1(velGnd) -> velGnd/1
  sMatrix_IP_LVDT/1(IP_LVDT) -> IP_LVDT/1
  sMatrix_GAS_LVDT/1(GAS_LVDT) -> GAS_LVDT/1
  sMatrix_BF_LVDT/1(BF_LVDT) -> BF_LVDT/1
  Suspension/13(dispTM) -> dispTM/1, sMatrix_TM_OpLev/1(dispTM), sMatrix_TM_PS/2(dispTM)
  accGnd/1 -> Suspension/1(accGnd)
  actIP/1 -> Suspension/2(actIP)
  actGAS/1 -> aMatrix_GAS/1(aMat_in)
  actBF/1 -> aMatrix_BF/1(aMat_in)
  sMatrix_TM_OpLev/1(TM_OpLev) -> TM_OpLev/1
  aMatrix_GAS/1(actGAS) -> Suspension/3(actGAS)
  aMatrix_BF/1(actBF) -> Suspension/4(actBF)
  Suspension/7(dispPF) -> sMatrix_PF_OpLev/1(dispPF)
  sMatrix_PF_OpLev/1(OpLev_PF) -> PF_OpLev/1
  Suspension/8(dispMNR) -> sMatrix_MN_PS/1(dispMNR)
  Suspension/9(dispMN) -> sMatrix_MN_PS/2(dispMN), sMatrix_MN_OpLev/1(dispMN)
  sMatrix_MN_PS/1(MN_PS) -> MN_PS/1
  sMatrix_MN_OpLev/1(MN_OpLev) -> MN_OpLev/1
  Suspension/10(dispIR) -> sMatrix_IM_PS/1(dispIR)
  Suspension/11(dispIM) -> sMatrix_IM_PS/2(dispIM)
  sMatrix_IM_PS/1(IM_PS) -> IM_PS/1
  Suspension/12(dispRM) -> sMatrix_TM_PS/1(dispRM)
  sMatrix_TM_PS/1(TM_PS) -> TM_PS/1
  Suspension/14(velTM) -> velTM/1
  aMatrix_MN/1(actMNR) -> Sum1/2
  aMatrix_MN/2(actMN) -> Suspension/6(actMN)
  actMN/1 -> aMatrix_MN/1(aMat_in)
  actIM/1 -> aMatrix_IM/1(aMat_in)
  aMatrix_IM/1(actIR) -> Suspension/7(actIR)
  aMatrix_IM/2(actIM) -> Suspension/8(actIM)
  actTM/1 -> aMatrix_TM/1(aMat_in)
  aMatrix_TM/1(actRM) -> Suspension/9(actRM)
  Sum/1 -> Suspension/10(actTM)
  aMatrix_TM/2(actTM) -> Sum/1
  forceTM/1 -> Sum/2
  Suspension/3(velIP) -> IP_GEO/1
  Sum1/1 -> Suspension/5(actMNR)
  forceMNR/1 -> Sum1/1

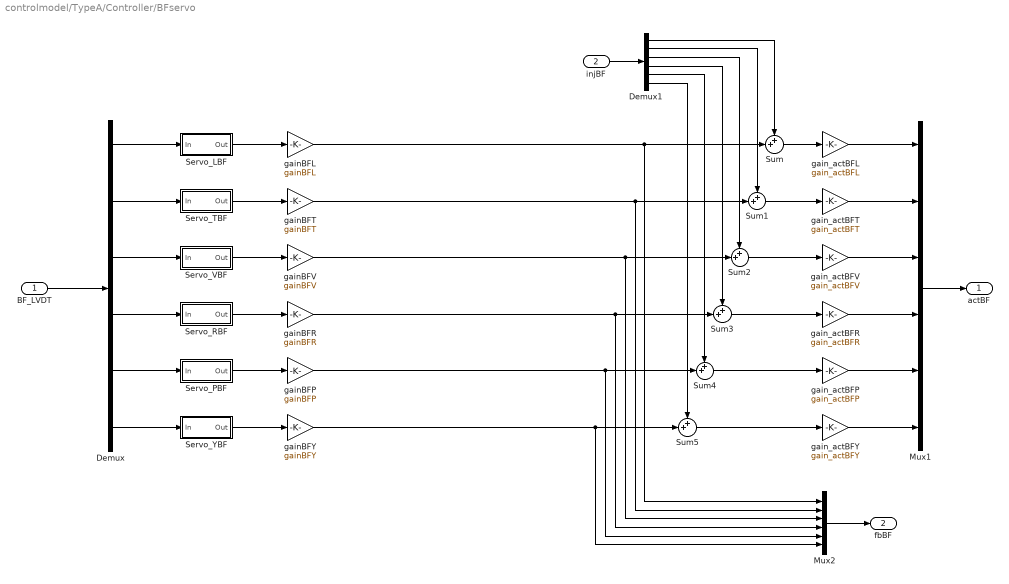
== system controlmodel/TypeA/Controller/BFservo ==
  BF_LVDT : Inport
  injBF : Inport  Port=2
  Demux : Demux  Outputs=6
  Demux1 : Demux  Outputs=6
  Mux1 : Mux  Inputs=6
  Mux2 : Mux  Inputs=6
  Servo_LBF : Subsystem
  Servo_PBF : Subsystem
  Servo_RBF : Subsystem
  Servo_TBF : Subsystem
  Servo_VBF : Subsystem
  Servo_YBF : Subsystem
  Sum{,1..5} (6 alike) : Sum  Inputs=++|
  gainBFL : Gain  Gain=gainBFL
  gainBFP : Gain  Gain=gainBFP
  gainBFR : Gain  Gain=gainBFR
  gainBFT : Gain  Gain=gainBFT
  gainBFV : Gain  Gain=gainBFV
  gainBFY : Gain  Gain=gainBFY
  gain_actBFL : Gain  Gain=gain_actBFL
  gain_actBFP : Gain  Gain=gain_actBFP
  gain_actBFR : Gain  Gain=gain_actBFR
  gain_actBFT : Gain  Gain=gain_actBFT
  gain_actBFV : Gain  Gain=gain_actBFV
  gain_actBFY : Gain  Gain=gain_actBFY
  actBF : Outport
  fbBF : Outport  Port=2
  wires:
  BF_LVDT/1 -> Demux/1
  Servo_LBF/1(Out) -> gainBFL/1
  Servo_TBF/1(Out) -> gainBFT/1
  Servo_VBF/1(Out) -> gainBFV/1
  Demux/1 -> Servo_LBF/1(In)
  Demux/2 -> Servo_TBF/1(In)
  Demux/3 -> Servo_VBF/1(In)
  gainBFL/1 -> Sum/2, Mux2/1
  gainBFT/1 -> Sum1/2, Mux2/2
  gainBFV/1 -> Sum2/2, Mux2/3
  injBF/1 -> Demux1/1
  Sum1/1 -> gain_actBFT/1
  Sum2/1 -> gain_actBFV/1
  Sum/1 -> gain_actBFL/1
  Mux1/1 -> actBF/1
  Mux2/1 -> fbBF/1
  Demux1/3 -> Sum2/1
  Demux1/2 -> Sum1/1
  Demux1/1 -> Sum/1
  Servo_RBF/1(Out) -> gainBFR/1
  Servo_PBF/1(Out) -> gainBFP/1
  gainBFR/1 -> Sum3/2, Mux2/4
  gainBFP/1 -> Sum4/2, Mux2/5
  Demux/4 -> Servo_RBF/1(In)
  Demux/5 -> Servo_PBF/1(In)
  Demux1/4 -> Sum3/1
  Demux1/5 -> Sum4/1
  Sum3/1 -> gain_actBFR/1
  Sum4/1 -> gain_actBFP/1
  Servo_YBF/1(Out) -> gainBFY/1
  gainBFY/1 -> Sum5/2, Mux2/6
  Demux/6 -> Servo_YBF/1(In)
  Sum5/1 -> gain_actBFY/1
  Demux1/6 -> Sum5/1
  gain_actBFV/1 -> Mux1/3
  gain_actBFY/1 -> Mux1/6
  gain_actBFR/1 -> Mux1/4
  gain_actBFT/1 -> Mux1/2
  gain_actBFL/1 -> Mux1/1
  gain_actBFP/1 -> Mux1/5

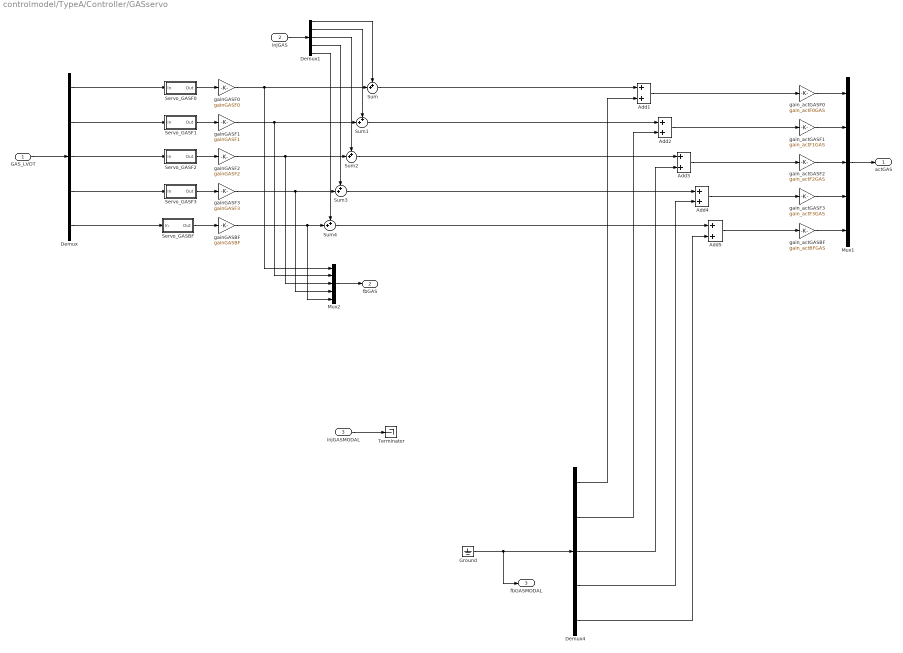
== system controlmodel/TypeA/Controller/GASservo ==
  GAS_LVDT : Inport
  injGAS : Inport  Port=2
  injGASMODAL : Inport  Port=3
  Add{1..5} (5 alike) : Sum
  Demux : Demux  Outputs=5
  Demux1 : Demux  Outputs=5
  Demux4 : Demux  Outputs=5
  Ground : Ground
  Mux1 : Mux  Inputs=5
  Mux2 : Mux  Inputs=5
  Servo_GASBF : Subsystem
  Servo_GASF0 : Subsystem
  Servo_GASF1 : Subsystem
  Servo_GASF2 : Subsystem
  Servo_GASF3 : Subsystem
  Sum{,1..4} (5 alike) : Sum  Inputs=++|
  Terminator : Terminator
  gainGASBF : Gain  Gain=gainGASBF
  gainGASF0 : Gain  Gain=gainGASF0
  gainGASF1 : Gain  Gain=gainGASF1
  gainGASF2 : Gain  Gain=gainGASF2
  gainGASF3 : Gain  Gain=gainGASF3
  gain_actGASBF : Gain  Gain=gain_actBFGAS
  gain_actGASF0 : Gain  Gain=gain_actF0GAS
  gain_actGASF1 : Gain  Gain=gain_actF1GAS
  gain_actGASF2 : Gain  Gain=gain_actF2GAS
  gain_actGASF3 : Gain  Gain=gain_actF3GAS
  actGAS : Outport
  fbGAS : Outport  Port=2
  fbGASMODAL : Outport  Port=3
  wires:
  GAS_LVDT/1 -> Demux/1
  Servo_GASF0/1(Out) -> gainGASF0/1
  Servo_GASF1/1(Out) -> gainGASF1/1
  Servo_GASF2/1(Out) -> gainGASF2/1
  Demux/1 -> Servo_GASF0/1(In)
  Demux/2 -> Servo_GASF1/1(In)
  Demux/3 -> Servo_GASF2/1(In)
  gainGASF0/1 -> Sum/2, Mux2/1
  gainGASF1/1 -> Sum1/2, Mux2/2
  gainGASF2/1 -> Sum2/2, Mux2/3
  injGAS/1 -> Demux1/1
  Mux1/1 -> actGAS/1
  Mux2/1 -> fbGAS/1
  Demux1/3 -> Sum2/1
  Demux1/2 -> Sum1/1
  Demux1/1 -> Sum/1
  Servo_GASF3/1(Out) -> gainGASF3/1
  Servo_GASBF/1(Out) -> gainGASBF/1
  gainGASF3/1 -> Sum3/2, Mux2/4
  gainGASBF/1 -> Sum4/2, Mux2/5
  Demux/4 -> Servo_GASF3/1(In)
  Demux/5 -> Servo_GASBF/1(In)
  Demux1/4 -> Sum3/1
  Demux1/5 -> Sum4/1
  gain_actGASF0/1 -> Mux1/1
  gain_actGASF2/1 -> Mux1/3
  gain_actGASF1/1 -> Mux1/2
  gain_actGASF3/1 -> Mux1/4
  gain_actGASBF/1 -> Mux1/5
  Ground/1 -> fbGASMODAL/1, Demux4/1
  Sum/1 -> Add1/1
  Add1/1 -> gain_actGASF0/1
  Add3/1 -> gain_actGASF2/1
  Sum2/1 -> Add3/1
  Add2/1 -> gain_actGASF1/1
  Sum1/1 -> Add2/1
  Sum3/1 -> Add4/1
  Add4/1 -> gain_actGASF3/1
  Add5/1 -> gain_actGASBF/1
  Sum4/1 -> Add5/1
  Demux4/1 -> Add1/2
  Demux4/2 -> Add2/2
  Demux4/3 -> Add3/2
  Demux4/4 -> Add4/2
  Demux4/5 -> Add5/2
  injGASMODAL/1 -> Terminator/1

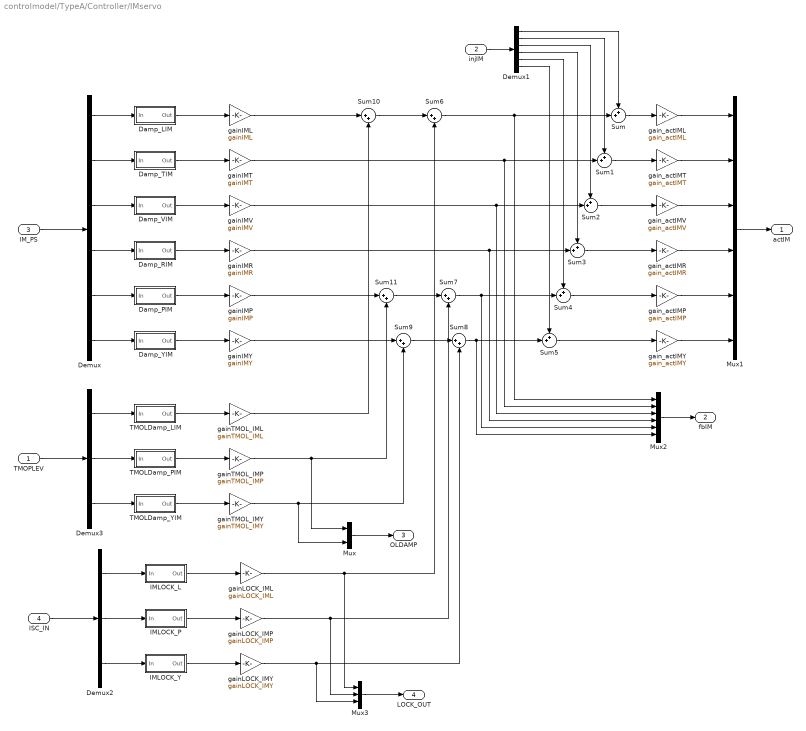
== system controlmodel/TypeA/Controller/IMservo ==
  TMOPLEV : Inport
  injIM : Inport  Port=2
  IM_PS : Inport  Port=3
  ISC_IN : Inport  Port=4
  Damp_LIM : Subsystem
  Damp_PIM : Subsystem
  Damp_RIM : Subsystem
  Damp_TIM : Subsystem
  Damp_VIM : Subsystem
  Damp_YIM : Subsystem
  Demux : Demux  Outputs=6
  Demux1 : Demux  Outputs=6
  Demux2 : Demux  Outputs=3
  Demux3 : Demux  Outputs=3
  IMLOCK_L : Subsystem
  IMLOCK_P : Subsystem
  IMLOCK_Y : Subsystem
  Mux : Mux  Inputs=2
  Mux1 : Mux  Inputs=6
  Mux2 : Mux  Inputs=6
  Mux3 : Mux  Inputs=3
  Sum{,1..5} (6 alike) : Sum  Inputs=++|
  Sum{6..11} (6 alike) : Sum  Inputs=|++
  TMOLDamp_LIM : Subsystem
  TMOLDamp_PIM : Subsystem
  TMOLDamp_YIM : Subsystem
  gainIML : Gain  Gain=gainIML
  gainIMP : Gain  Gain=gainIMP
  gainIMR : Gain  Gain=gainIMR
  gainIMT : Gain  Gain=gainIMT
  gainIMV : Gain  Gain=gainIMV
  gainIMY : Gain  Gain=gainIMY
  gainLOCK_IML : Gain  Gain=gainLOCK_IML
  gainLOCK_IMP : Gain  Gain=gainLOCK_IMP
  gainLOCK_IMY : Gain  Gain=gainLOCK_IMY
  gainTMOL_IML : Gain  Gain=gainTMOL_IML
  gainTMOL_IMP : Gain  Gain=gainTMOL_IMP
  gainTMOL_IMY : Gain  Gain=gainTMOL_IMY
  gain_actIML : Gain  Gain=gain_actIML
  gain_actIMP : Gain  Gain=gain_actIMP
  gain_actIMR : Gain  Gain=gain_actIMR
  gain_actIMT : Gain  Gain=gain_actIMT
  gain_actIMV : Gain  Gain=gain_actIMV
  gain_actIMY : Gain  Gain=gain_actIMY
  actIM : Outport
  fbIM : Outport  Port=2
  OLDAMP : Outport  Port=3
  LOCK_OUT : Outport  Port=4
  wires:
  injIM/1 -> Demux1/1
  Sum1/1 -> gain_actIMT/1
  Sum2/1 -> gain_actIMV/1
  Sum/1 -> gain_actIML/1
  Mux1/1 -> actIM/1
  Mux2/1 -> fbIM/1
  Demux1/3 -> Sum2/1
  Demux1/2 -> Sum1/1
  Demux1/1 -> Sum/1
  Demux1/4 -> Sum3/1
  Demux1/5 -> Sum4/1
  Sum3/1 -> gain_actIMR/1
  Sum4/1 -> gain_actIMP/1
  Sum5/1 -> gain_actIMY/1
  Demux1/6 -> Sum5/1
  gain_actIMV/1 -> Mux1/3
  gain_actIMY/1 -> Mux1/6
  gain_actIMR/1 -> Mux1/4
  gain_actIMT/1 -> Mux1/2
  gain_actIML/1 -> Mux1/1
  gain_actIMP/1 -> Mux1/5
  TMOLDamp_LIM/1(Out) -> gainTMOL_IML/1
  TMOLDamp_PIM/1(Out) -> gainTMOL_IMP/1
  TMOLDamp_YIM/1(Out) -> gainTMOL_IMY/1
  TMOPLEV/1 -> Demux3/1
  Demux3/1 -> TMOLDamp_LIM/1(In)
  Demux3/2 -> TMOLDamp_PIM/1(In)
  Demux3/3 -> TMOLDamp_YIM/1(In)
  gainTMOL_IML/1 -> Sum10/2
  gainTMOL_IMP/1 -> Mux/1, Sum11/2
  gainTMOL_IMY/1 -> Mux/2, Sum9/2
  IM_PS/1 -> Demux/1
  Damp_LIM/1(Out) -> gainIML/1
  Damp_TIM/1(Out) -> gainIMT/1
  Damp_VIM/1(Out) -> gainIMV/1
  Demux/1 -> Damp_LIM/1(In)
  Demux/2 -> Damp_TIM/1(In)
  Demux/3 -> Damp_VIM/1(In)
  Damp_RIM/1(Out) -> gainIMR/1
  Damp_PIM/1(Out) -> gainIMP/1
  Demux/4 -> Damp_RIM/1(In)
  Demux/5 -> Damp_PIM/1(In)
  Damp_YIM/1(Out) -> gainIMY/1
  Demux/6 -> Damp_YIM/1(In)
  gainIML/1 -> Sum10/1
  gainIMT/1 -> Mux2/2, Sum1/2
  gainIMV/1 -> Mux2/3, Sum2/2
  gainIMR/1 -> Mux2/4, Sum3/2
  gainIMP/1 -> Sum11/1
  gainIMY/1 -> Sum9/1
  Mux/1 -> OLDAMP/1
  IMLOCK_L/1(Out) -> gainLOCK_IML/1
  IMLOCK_P/1(Out) -> gainLOCK_IMP/1
  IMLOCK_Y/1(Out) -> gainLOCK_IMY/1
  ISC_IN/1 -> Demux2/1
  Demux2/1 -> IMLOCK_L/1(In)
  Demux2/2 -> IMLOCK_P/1(In)
  Demux2/3 -> IMLOCK_Y/1(In)
  gainLOCK_IML/1 -> Mux3/1, Sum6/2
  gainLOCK_IMP/1 -> Mux3/2, Sum7/2
  gainLOCK_IMY/1 -> Mux3/3, Sum8/2
  Mux3/1 -> LOCK_OUT/1
  Sum10/1 -> Sum6/1
  Sum6/1 -> Mux2/1, Sum/2
  Sum9/1 -> Sum8/1
  Sum8/1 -> Mux2/6, Sum5/2
  Sum11/1 -> Sum7/1
  Sum7/1 -> Mux2/5, Sum4/2

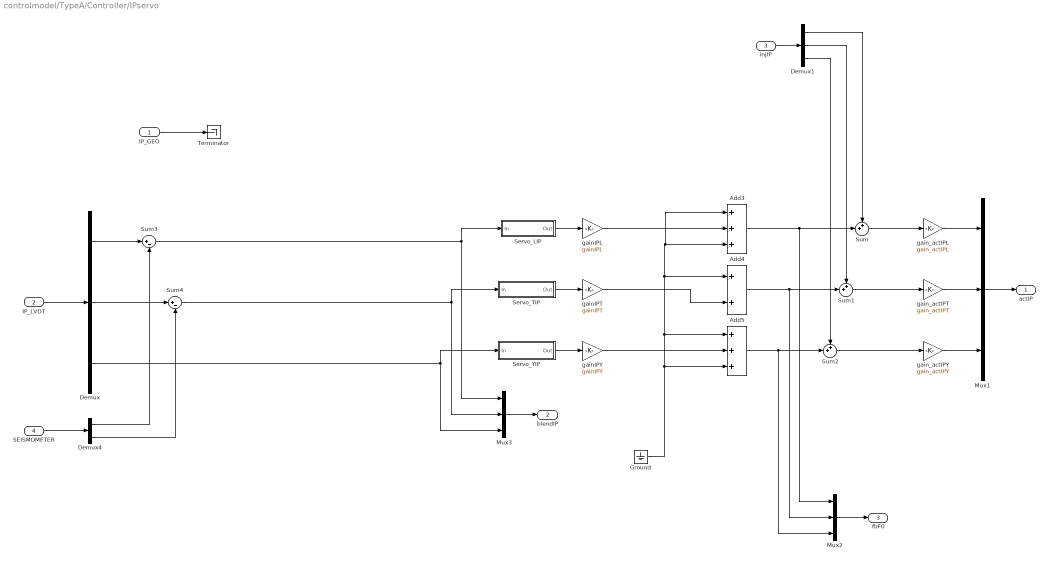
== system controlmodel/TypeA/Controller/IPservo ==
  IP_GEO : Inport
  IP_LVDT : Inport  Port=2
  injIP : Inport  Port=3
  SEISMOMETER : Inport  Port=4
  Add3 : Sum  Inputs=+++
  Add4 : Sum
  Add5 : Sum  Inputs=+++
  Demux : Demux  Outputs=3
  Demux1 : Demux  Outputs=3
  Demux4 : Demux  Outputs=2
  Ground : Ground
  Mux1 : Mux  Inputs=3
  Mux2 : Mux  Inputs=3
  Mux3 : Mux  Inputs=3
  Servo_LIP : Subsystem
  Servo_TIP : Subsystem
  Servo_YIP : Subsystem
  Sum : Sum  Inputs=++|
  Sum1 : Sum  Inputs=++|
  Sum2 : Sum  Inputs=++|
  Sum3 : Sum  Inputs=|+-
  Sum4 : Sum  Inputs=|+-
  Terminator : Terminator
  gainIPL : Gain  Gain=gainIPL
  gainIPT : Gain  Gain=gainIPT
  gainIPY : Gain  Gain=gainIPY
  gain_actIPL : Gain  Gain=gain_actIPL
  gain_actIPT : Gain  Gain=gain_actIPT
  gain_actIPY : Gain  Gain=gain_actIPY
  actIP : Outport
  blendIP : Outport  Port=2
  fbF0 : Outport  Port=3
  wires:
  IP_LVDT/1 -> Demux/1
  Servo_LIP/1(Out) -> gainIPL/1
  Servo_TIP/1(Out) -> gainIPT/1
  Servo_YIP/1(Out) -> gainIPY/1
  Add3/1 -> Sum/2, Mux2/1
  Add4/1 -> Sum1/2, Mux2/2
  Add5/1 -> Sum2/2, Mux2/3
  injIP/1 -> Demux1/1
  Sum1/1 -> gain_actIPT/1
  Sum2/1 -> gain_actIPY/1
  Sum/1 -> gain_actIPL/1
  Mux1/1 -> actIP/1
  Mux2/1 -> fbF0/1
  Demux1/3 -> Sum2/1
  Demux1/2 -> Sum1/1
  Demux1/1 -> Sum/1
  gain_actIPT/1 -> Mux1/2
  gain_actIPL/1 -> Mux1/1
  gain_actIPY/1 -> Mux1/3
  IP_GEO/1 -> Terminator/1
  Sum3/1 -> Servo_LIP/1(In), Mux3/1
  Sum4/1 -> Servo_TIP/1(In), Mux3/2
  Demux/3 -> Servo_YIP/1(In), Mux3/3
  Mux3/1 -> blendIP/1
  gainIPY/1 -> Add5/2
  gainIPT/1 -> Add4/2
  gainIPL/1 -> Add3/2
  SEISMOMETER/1 -> Demux4/1
  Demux/1 -> Sum3/1
  Demux/2 -> Sum4/1
  Demux4/1 -> Sum3/2
  Demux4/2 -> Sum4/2
  Ground/1 -> Add5/3, Add3/1, Add3/3, Add4/1, Add5/1

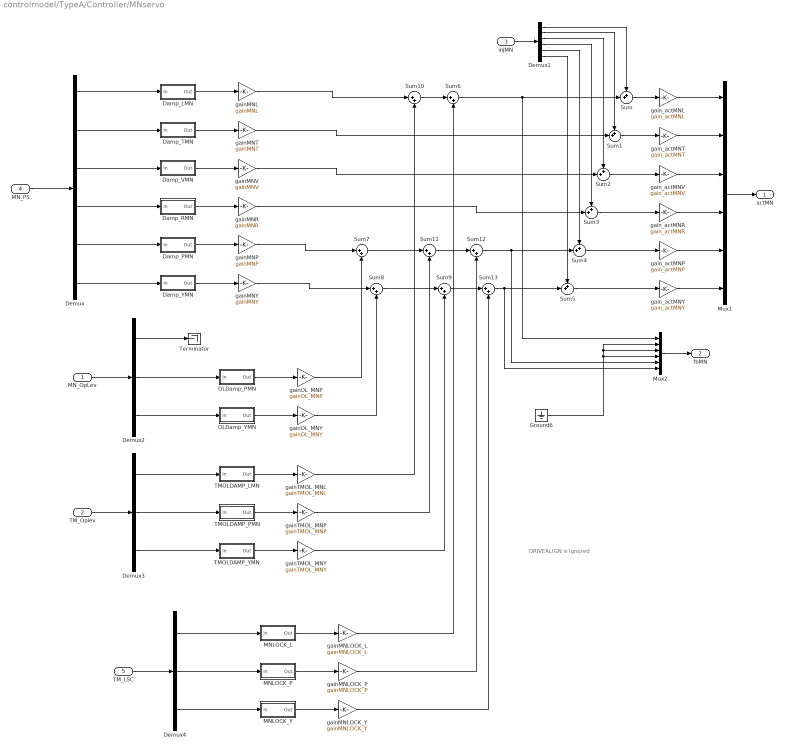
== system controlmodel/TypeA/Controller/MNservo ==
  note: DRIVEALIGN is Ignored
  MN_OpLev : Inport
  TM_Oplev : Inport  Port=2
  injMN : Inport  Port=3
  MN_PS : Inport  Port=4
  TM_LSC : Inport  Port=5
  Damp_LMN : Subsystem
  Damp_PMN : Subsystem
  Damp_RMN : Subsystem
  Damp_TMN : Subsystem
  Damp_VMN : Subsystem
  Damp_YMN : Subsystem
  Demux : Demux  Outputs=6
  Demux1 : Demux  Outputs=6
  Demux2 : Demux  Outputs=3
  Demux3 : Demux  Outputs=3
  Demux4 : Demux  Outputs=3
  Ground6 : Ground
  MNLOCK_L : Subsystem
  MNLOCK_P : Subsystem
  MNLOCK_Y : Subsystem
  Mux1 : Mux  Inputs=6
  Mux2 : Mux  Inputs=6
  OLDamp_PMN : Subsystem
  OLDamp_YMN : Subsystem
  Sum{,1..5} (6 alike) : Sum  Inputs=++|
  Sum{6..13} (8 alike) : Sum  Inputs=|++
  TMOLDAMP_LMN : Subsystem
  TMOLDAMP_PMN : Subsystem
  TMOLDAMP_YMN : Subsystem
  Terminator : Terminator
  gainMNL : Gain  Gain=gainMNL
  gainMNLOCK_L : Gain  Gain=gainMNLOCK_L
  gainMNLOCK_P : Gain  Gain=gainMNLOCK_P
  gainMNLOCK_Y : Gain  Gain=gainMNLOCK_Y
  gainMNP : Gain  Gain=gainMNP
  gainMNR : Gain  Gain=gainMNR
  gainMNT : Gain  Gain=gainMNT
  gainMNV : Gain  Gain=gainMNV
  gainMNY : Gain  Gain=gainMNY
  gainOL_MNP : Gain  Gain=gainOL_MNP
  gainOL_MNY : Gain  Gain=gainOL_MNY
  gainTMOL_MNL : Gain  Gain=gainTMOL_MNL
  gainTMOL_MNP : Gain  Gain=gainTMOL_MNP
  gainTMOL_MNY : Gain  Gain=gainTMOL_MNY
  gain_actMNL : Gain  Gain=gain_actMNL
  gain_actMNP : Gain  Gain=gain_actMNP
  gain_actMNR : Gain  Gain=gain_actMNR
  gain_actMNT : Gain  Gain=gain_actMNT
  gain_actMNV : Gain  Gain=gain_actMNV
  gain_actMNY : Gain  Gain=gain_actMNY
  actMN : Outport
  fbMN : Outport  Port=2
  wires:
  injMN/1 -> Demux1/1
  Sum1/1 -> gain_actMNT/1
  Sum2/1 -> gain_actMNV/1
  Sum/1 -> gain_actMNL/1
  Mux1/1 -> actMN/1
  Mux2/1 -> fbMN/1
  Demux1/3 -> Sum2/1
  Demux1/2 -> Sum1/1
  Demux1/1 -> Sum/1
  Demux1/4 -> Sum3/1
  Demux1/5 -> Sum4/1
  Sum3/1 -> gain_actMNR/1
  Sum4/1 -> gain_actMNP/1
  Sum5/1 -> gain_actMNY/1
  Demux1/6 -> Sum5/1
  gain_actMNV/1 -> Mux1/3
  gain_actMNY/1 -> Mux1/6
  gain_actMNR/1 -> Mux1/4
  gain_actMNT/1 -> Mux1/2
  gain_actMNL/1 -> Mux1/1
  gain_actMNP/1 -> Mux1/5
  TMOLDAMP_LMN/1(Out) -> gainTMOL_MNL/1
  TMOLDAMP_PMN/1(Out) -> gainTMOL_MNP/1
  TMOLDAMP_YMN/1(Out) -> gainTMOL_MNY/1
  OLDamp_PMN/1(Out) -> gainOL_MNP/1
  OLDamp_YMN/1(Out) -> gainOL_MNY/1
  MN_OpLev/1 -> Demux2/1
  TM_Oplev/1 -> Demux3/1
  Demux2/2 -> OLDamp_PMN/1(In)
  Demux2/3 -> OLDamp_YMN/1(In)
  Demux3/1 -> TMOLDAMP_LMN/1(In)
  gainOL_MNP/1 -> Sum7/2
  gainOL_MNY/1 -> Sum8/2
  Sum7/1 -> Sum11/1
  gainTMOL_MNL/1 -> Sum10/2
  gainTMOL_MNP/1 -> Sum11/2
  gainTMOL_MNY/1 -> Sum9/2
  Sum8/1 -> Sum9/1
  Demux3/2 -> TMOLDAMP_PMN/1(In)
  Demux3/3 -> TMOLDAMP_YMN/1(In)
  Demux2/1 -> Terminator/1
  gainMNL/1 -> Sum10/1
  gainMNT/1 -> Sum1/2
  gainMNV/1 -> Sum2/2
  gainMNR/1 -> Sum3/2
  Ground6/1 -> Mux2/4, Mux2/3, Mux2/2
  MN_PS/1 -> Demux/1
  Damp_LMN/1(Out) -> gainMNL/1
  Damp_TMN/1(Out) -> gainMNT/1
  Damp_VMN/1(Out) -> gainMNV/1
  Demux/1 -> Damp_LMN/1(In)
  Demux/2 -> Damp_TMN/1(In)
  Demux/3 -> Damp_VMN/1(In)
  Damp_RMN/1(Out) -> gainMNR/1
  Damp_PMN/1(Out) -> gainMNP/1
  Demux/4 -> Damp_RMN/1(In)
  Demux/5 -> Damp_PMN/1(In)
  Damp_YMN/1(Out) -> gainMNY/1
  Demux/6 -> Damp_YMN/1(In)
  gainMNP/1 -> Sum7/1
  gainMNY/1 -> Sum8/1
  MNLOCK_L/1(Out) -> gainMNLOCK_L/1
  MNLOCK_P/1(Out) -> gainMNLOCK_P/1
  MNLOCK_Y/1(Out) -> gainMNLOCK_Y/1
  TM_LSC/1 -> Demux4/1
  Demux4/1 -> MNLOCK_L/1(In)
  gainMNLOCK_L/1 -> Sum6/2
  gainMNLOCK_P/1 -> Sum12/2
  gainMNLOCK_Y/1 -> Sum13/2
  Demux4/2 -> MNLOCK_P/1(In)
  Demux4/3 -> MNLOCK_Y/1(In)
  Sum10/1 -> Sum6/1
  Sum6/1 -> Mux2/1, Sum/2
  Sum12/1 -> Mux2/5, Sum4/2
  Sum11/1 -> Sum12/1
  Sum9/1 -> Sum13/1
  Sum13/1 -> Mux2/6, Sum5/2

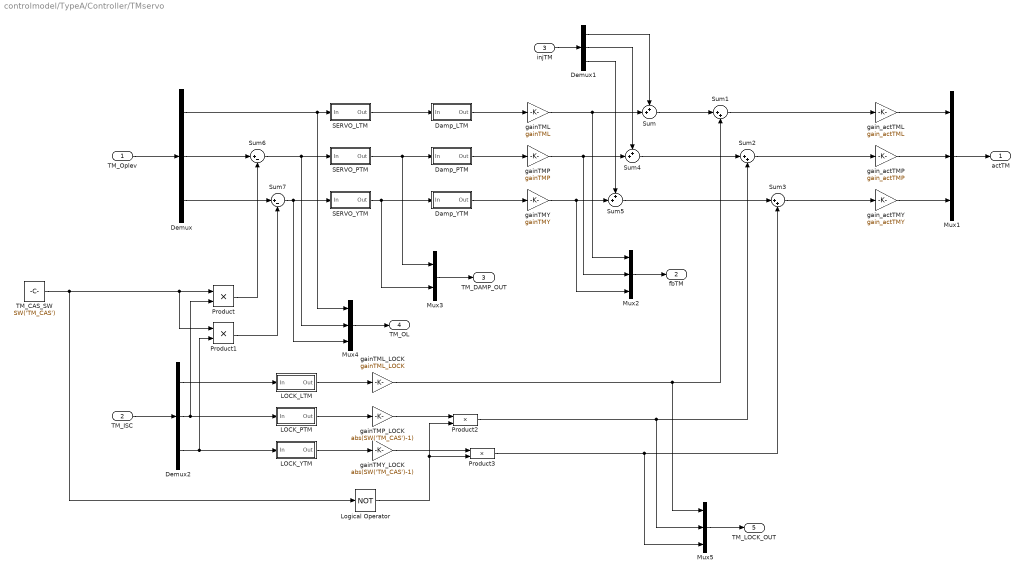
== system controlmodel/TypeA/Controller/TMservo ==
  TM_Oplev : Inport
  TM_ISC : Inport  Port=2
  injTM : Inport  Port=3
  Damp_LTM : Subsystem
  Damp_PTM : Subsystem
  Damp_YTM : Subsystem
  Demux : Demux  Outputs=3
  Demux1 : Demux  Outputs=3
  Demux2 : Demux  Outputs=3
  LOCK_LTM : Subsystem
  LOCK_PTM : Subsystem
  LOCK_YTM : Subsystem
  Logical Operator : Logic  Operator=NOT  Inputs=1  AllPortsSameDT=off  OutDataTypeStr=boolean
  Mux{1..2,4..5} (4 alike) : Mux  Inputs=3
  Mux3 : Mux  Inputs=2
  Product{,1..3} (4 alike) : Product
  SERVO_LTM : Subsystem
  SERVO_PTM : Subsystem
  SERVO_YTM : Subsystem
  Sum : Sum  Inputs=++|
  Sum1 : Sum  Inputs=|++
  Sum2 : Sum  Inputs=|++
  Sum3 : Sum  Inputs=|++
  Sum4 : Sum  Inputs=++|
  Sum5 : Sum  Inputs=++|
  Sum6 : Sum  Inputs=|+-
  Sum7 : Sum  Inputs=|+-
  TM_CAS_SW : Constant  Value=SW('TM_CAS')
  gainTML : Gain  Gain=gainTML
  gainTML_LOCK : Gain  Gain=gainTML_LOCK
  gainTMP : Gain  Gain=gainTMP
  gainTMP_LOCK : Gain  Gain=abs(SW('TM_CAS')-1)
  gainTMY : Gain  Gain=gainTMY
  gainTMY_LOCK : Gain  Gain=abs(SW('TM_CAS')-1)
  gain_actTML : Gain  Gain=gain_actTML
  gain_actTMP : Gain  Gain=gain_actTMP
  gain_actTMY : Gain  Gain=gain_actTMY
  actTM : Outport
  fbTM : Outport  Port=2
  TM_DAMP_OUT : Outport  Port=3
  TM_OL : Outport  Port=4
  TM_LOCK_OUT : Outport  Port=5
  wires:
  TM_Oplev/1 -> Demux/1
  Damp_LTM/1(Out) -> gainTML/1
  gainTML/1 -> Sum/2, Mux2/1
  injTM/1 -> Demux1/1
  Mux1/1 -> actTM/1
  Mux2/1 -> fbTM/1
  Demux1/1 -> Sum/1
  Damp_PTM/1(Out) -> gainTMP/1
  gainTMP/1 -> Mux2/2, Sum4/2
  Damp_YTM/1(Out) -> gainTMY/1
  gainTMY/1 -> Mux2/3, Sum5/2
  gain_actTML/1 -> Mux1/1
  Demux1/2 -> Sum4/1
  Demux1/3 -> Sum5/1
  gain_actTMP/1 -> Mux1/2
  gain_actTMY/1 -> Mux1/3
  TM_ISC/1 -> Demux2/1
  SERVO_PTM/1(Out) -> Mux3/1, Damp_PTM/1(In)
  SERVO_YTM/1(Out) -> Mux3/2, Damp_YTM/1(In)
  Mux3/1 -> TM_DAMP_OUT/1
  Demux2/1 -> LOCK_LTM/1(In)
  Demux2/2 -> Product/2, LOCK_PTM/1(In)
  Demux2/3 -> Product1/2, LOCK_YTM/1(In)
  SERVO_LTM/1(Out) -> Damp_LTM/1(In)
  LOCK_LTM/1(Out) -> gainTML_LOCK/1
  LOCK_PTM/1(Out) -> gainTMP_LOCK/1
  LOCK_YTM/1(Out) -> gainTMY_LOCK/1
  Sum/1 -> Sum1/1
  Sum1/1 -> gain_actTML/1
  Sum4/1 -> Sum2/1
  Sum2/1 -> gain_actTMP/1
  Sum5/1 -> Sum3/1
  Sum3/1 -> gain_actTMY/1
  TM_CAS_SW/1 -> Logical Operator/1, Product/1, Product1/1
  Demux/2 -> Sum6/1
  Demux/3 -> Sum7/1
  Sum7/1 -> Mux4/3, SERVO_YTM/1(In)
  Product/1 -> Sum6/2
  Product1/1 -> Sum7/2
  Demux/1 -> Mux4/1, SERVO_LTM/1(In)
  Sum6/1 -> Mux4/2, SERVO_PTM/1(In)
  Mux4/1 -> TM_OL/1
  gainTMP_LOCK/1 -> Product2/1
  Logical Operator/1 -> Product3/2, Product2/2
  gainTMY_LOCK/1 -> Product3/1
  Product3/1 -> Mux5/3, Sum3/2
  gainTML_LOCK/1 -> Mux5/1, Sum1/2
  Product2/1 -> Mux5/2, Sum2/2
  Mux5/1 -> TM_LOCK_OUT/1
